simulink model "Furnace"  (R2020a)
settings: Solver=ode15s  StartTime=0  StopTime=27000  FixedStep=0.1  MaxStep=20  MinStep=1e-13  RelTol=1e-08  AbsTol=1e-09
undefined symbols (not defined in the file): agnostic_lqe_params, cont_reg, disturbance_type, F_aI_pid, F_aII_pid, input_type, k, lqe_params, LQR_params, LQRAgnostic_params, MPC_type, MPCDiscrete_function_parameters, MPCDiscreteAgnostic_function_parameters, MPCDiscreteDiffIntegralAgnostic_function_parameters, original_LQR_params, output_type, reg, single_butter_ss
libraries: simulink x35, cstblocks x10, mpclib x3
(part 7 of 8)

== matlab function Furnace/Controller/Input  selector1 ==
  data: constant input; signal output; experimental input; controlled input; input_type input
function signal = ChooseSignal(constant, experimental, controlled, input_type)
    switch(input_type)
        case InputType.Experimental
            signal = experimental;
        case InputType.Controlled
            signal = controlled;
        otherwise
            signal = constant;
    end
end

== matlab function Furnace/Controller/Input  selector2 ==
  data: constant input; signal output; experimental input; controlled input; input_type input
function signal = ChooseSignal(constant, experimental, controlled, input_type)
    switch(input_type)
        case InputType.Experimental
            signal = experimental;
        case InputType.Controlled
            signal = controlled;
        otherwise
            signal = constant;
    end
end

== matlab function Furnace/Controller/Input  selector5 ==
  data: constant input; signal output; experimental input; controlled input; input_type input
function signal = ChooseSignal(constant, experimental, controlled, input_type)
    switch(input_type)
        case InputType.Experimental
            signal = experimental;
        case InputType.Controlled
            signal = controlled;
        otherwise
            signal = constant;
    end
end

== matlab function Furnace/Actuator dynamics/Secondary air/Input  selector ==
  data: constant input; signal output; experimental input; step input; controlled input; input_type input
function signal = ChooseSignal(constant, experimental, step, controlled, input_type)
    switch(input_type)
        case InputType.Experimental
            signal = experimental;
        case InputType.Controlled
            signal = controlled;
        case InputType.Step
            signal = step; 
        otherwise
            signal = constant;
    end
end

== matlab function Furnace/Actuator dynamics/Secondary air/Input  selector1 ==
  data: constant input; signal output; experimental input; step input; controlled input; input_type input
function signal = ChooseSignal(constant, experimental, step, controlled, input_type)
    switch(input_type)
        case InputType.Experimental
            signal = experimental;
        case InputType.Controlled
            signal = controlled;
        case InputType.Step
            signal = step; 
        otherwise
            signal = constant;
    end
end

== matlab function Furnace/Actuator dynamics/Waste and Primary air/Input selector ==
  data: constant input; signal output; experimental input; controlled input; input_type input
function signal = ChooseSignal(constant, experimental, controlled, input_type)
    switch(input_type)
        case InputType.Experimental
            signal = experimental;
        case InputType.Controlled
            signal = controlled;
        otherwise
            signal = constant;
    end
end

== matlab function Furnace/Deprecated, slow loop/Furnace/Boiler/Economizer/Economizer ==
  data: Fi_fg input; F_w input; Q_ECO output; T_ECO input; T_fg2 input; cp_fg input; epsilon_ECO input; T_fg3 output; eff_HE input; cp_w input; T_ECO2 output
function [Q_ECO,T_fg3,T_ECO2] = CALC_Q_ECO(Fi_fg,F_w,T_ECO,T_fg2,cp_fg,epsilon_ECO,eff_HE, cp_w)

% This function calculates the heat exchanged in the economizer

F_fg    = sum(Fi_fg);
C_min   = cp_fg.*F_fg;
if F_w == 0 
    Q_ECO   = 0;
    T_fg3   = T_fg2;
    T_ECO2  = T_ECO;
else
    Q_ECO   = epsilon_ECO.*C_min.*(T_fg2-T_ECO);
    T_fg3   = T_fg2 - Q_ECO./(cp_fg.*F_fg);
    T_ECO2  = T_ECO + Q_ECO.*eff_HE./(cp_w.*F_w);
end
Q_ECO       = Q_ECO.*eff_HE;

== matlab function Furnace/Actuator dynamics/Waste and Primary air/Input  selector ==
  data: constant input; signal output; experimental input; step input; controlled input; input_type input
function signal = ChooseSignal(constant, experimental, step, controlled, input_type)
    switch(input_type)
        case InputType.Experimental
            signal = experimental;
        case InputType.Controlled
            signal = controlled;
        case InputType.Step
            signal = step; 
        otherwise
            signal = constant;
    end
end

== matlab function Furnace/Actuator dynamics/Waste and Primary air/Input  selector1 ==
  data: constant input; signal output; experimental input; step input; controlled input; input_type input
function signal = ChooseSignal(constant, experimental, step, controlled, input_type)
    switch(input_type)
        case InputType.Experimental
            signal = experimental;
        case InputType.Controlled
            signal = controlled;
        case InputType.Step
            signal = step; 
        otherwise
            signal = constant;
    end
end

== matlab function Furnace/Actuator dynamics/Grate speed/Input  selector ==
  data: constant input; signal output; experimental input; step input; controlled input; input_type input
function signal = ChooseSignal(constant, experimental, step, controlled, input_type)
    switch(input_type)
        case InputType.Experimental
            signal = experimental;
        case InputType.Controlled
            signal = controlled;
        case InputType.Step
            signal = step; 
        otherwise
            signal = constant;
    end
end

== matlab function Furnace/Actuator dynamics/Grate speed/Input  selector1 ==
  data: constant input; signal output; experimental input; step input; controlled input; input_type input
function signal = ChooseSignal(constant, experimental, step, controlled, input_type)
    switch(input_type)
        case InputType.Experimental
            signal = experimental;
        case InputType.Controlled
            signal = controlled;
        case InputType.Step
            signal = step; 
        otherwise
            signal = constant;
    end
end

== matlab function Furnace/Deprecated, slow loop/Furnace/Condenser/District heating heat exchanger ==
  data: F_DH input; Q_HE output; p_HP input; F_turb input; T_return input; cp_water input; epsilon_HE input; Tw_ECO output; T_district output; eff_HE input
function [Q_HE,Tw_ECO,T_district] = CALC_Q_HE(F_DH,p_HP,F_turb,T_return,cp_water,epsilon_HE,eff_HE)

% This function calculates the heat exchanged between the steam from the
% drum and the water from the district heating net
C_min   = cp_water.*F_DH;
[p_sat,T_sat,~,~,~,~] = SatWater;
T_HP    = interp1(p_sat,T_sat,p_HP,'linear','extrap');
if F_turb == 0
    Q_HE    = 0;
else 
    
    Q_HE    = epsilon_HE.*C_min.*(T_HP-T_return);
end
Tw_ECO      = T_HP;
T_district  = T_return + Q_HE./C_min;
Q_HE        = Q_HE./eff_HE;

== matlab function Furnace/Deprecated, slow loop/Furnace/Boiler/Drum/DIFF_Boiler  ==
  data: Q_EVA input; dA_dt output size=1; F_ECO input; F_SH input; T_ECO input; T_drum input; Q_cleaning input; cp_water input; dM_dt output
function [dA_dt,dM_dt]  = DIFF_Boiler(Q_EVA ,F_ECO, F_SH,T_ECO, T_drum, Q_cleaning,cp_water)

% Energy in the drum [J]
%% ENERGY BALANCE EQUATION
[~,T_sat,~,h_w,h_vap,~] = SatWater;
if T_drum < 373.15
    dA_dt   = Q_EVA - Q_cleaning;
    dM_dt   = 0;
else
    % Enthalpy of water vapor at T_drum [J/kg]
    h_steam = interp1(T_sat,h_vap,T_drum,'linear','extrap');
    % Enthalpy of water at T_drum [J/kg]
    h_water = interp1(T_sat,h_w,T_drum,'linear','extrap');
    h_ECO   = h_water - cp_water.*(T_drum-T_ECO);
    % Energy balance
    dA_dt   = Q_EVA - F_SH.*h_steam  + F_ECO.*h_ECO - Q_cleaning;
    dM_dt   = - F_SH + F_ECO;
end

== matlab function Furnace/Deprecated, slow loop/Furnace/Boiler/Drum/DIFF_Boiler_2 ==
  data: A input; T_drum output; p_amb input; T_amb input; Mw_water input; V_gas input; M_H2O input; cp_water input; V_EVA input; rho_water input; M_steel input; cp_steel input; cp_fg input; Mw_air input; p output
function [T_drum,p] = Boiler(A,p_amb,T_amb,Mw_water,V_gas,M_H2O,cp_water,V_EVA,rho_water,M_steel,cp_steel,cp_fg,Mw_air)

% This function calculates the pressure and temperature in the boiler drum
% from the total energy in the drum. The start up description should be
% changed when we know how boiler start up actually works.

%%%%%%%%%%%%%%%%%%%%%%%%%%%%%%%%%%%%%%%%%%%%%%%%%%%%%%%%%%%%%%%%%%%%%%%%%%%
% Symbol        Units       Explanation
% INPUTS:
% A             [J]         Energy stored in the boiler drum
% p_amb         [Pa]        Ambient pressure
% T_amb         [K]         Ambient temperature
% Mw_water      [kg/kmol]   Molar weight of water
% V_gas         [m3]        Volume of drum boiler initilly occupied by air
% M_H2O         [kg]        Mass of water in the boiler
% cp_water      [J/kg K]    Specific heat capacity of water
% V_EVA         [m3]        Total volume of boiler
% rho_water     [kg/m3]     Density of water
% M_steel       [kg]        Total mass of steel in the boiler
% cp_steel      [J/kg K]    Specific heat capacity of steel
% cp_fg         [J/kg K]    Specific heat capicity of fuel gasses
% Mw_air        [kg/kmol]   Molar weight of air/fuel gasses
%%%%%%%%%%%%%%%%%%%%%%%%%%%%%%%%%%%%%%%%%%%%%%%%%%%%%%%%%%%%%%%%%%%%%%%%%%%

% Energy in the drum [J]
A_en        = A;
R           = 8.314462175*1E3;
%% ENERGY BALANCE EQUATION
[p_sat,T_sat,rho_vap,h_w,h_vap,~] = SatWater;
T_drum      = fzero(@find_T,273);
if T_drum < 373.15
    p  	= p_amb;
else
    p   = interp1(T_sat,p_sat,T_drum,'linear','extrap');
end

%%%%%%%%%%%%%%%%%%%%%%%%%%%%%%%%%%%%%%%%%%%%%%%%%%%%%%%%%%%%%%%%%%%%%%%%%%%
% This subfunction finds the temperature of the drum that satisfies the
% energy balance. We assume that the cold boiler is initially filled with
% water (M_H2O) and air (which occupies the volume V_gas). The boiler has a
% valve, which is open as long as T_drum<373.15K, so that the air can be
% discharged in the atmosphere as the boiler warms up and the water
% eveporates. In this way, the pressure is mantained at p=p_amb. When
% T_drum reaches 373.15K, the valve closes and pressure builds up as the
% water starts evaporating, so that saturated water and steam are always
% present in the vessel, at the relative saturated temperature and pressure

    function Res    = find_T(X)
        T_drum      = X;
        if T_drum < 373.15
            % When T_drum<375.15K, the valve is open and p=p_amb [Pa]
            p       = p_amb;
            % The air is assumed to be saturated with water [kmol_vap/kmol]
            y_sat   = CALC_xsat(T_drum);
            % Partial pressure of water vapor [Pa]
            p_vap   = y_sat*p;
            % Specific entalphy of water at 373.15K [J/kg]
            h_w_sat = interp1(T_sat,h_w,373.15,'linear','extrap');
            % Enthalpy of water at T_drum [J/kg]
            h_water = h_w_sat - cp_water.*(373.15-T_drum);
            % Enthalpy of water vapor at T_drum [J/kg]
            h_steam = interp1(T_sat,h_vap,T_drum,'linear','extrap');
            % Vapor fraction
            x_vap   = fzero(@find_x_vap,0);
            % Moles of air in the drum [kmol]
            N_air   = (p-p_vap).*V_gas./(R.*T_drum);
            % Mass of air in the drum [kg]
            M_air   = N_air.*Mw_air;
        else
            % Enthalpy of water vapor at T_drum [J/kg]
            h_steam = interp1(T_sat,h_vap,T_drum,'linear','extrap');
            % Enthalpy of water at T_drum [J/kg]
            h_water = interp1(T_sat,h_w,T_drum,'linear','extrap');
            % Pressure of boiling water at T_drum [Pa]
            p       = interp1(T_sat,p_sat,T_drum,'linear','extrap');
            % Find the vapor fraction
            x_vap   = fzero(@find_x_vap,0);
            % No air is left in the boiler after start up
            M_air   = 0;
        end

        Res         = A_en- (M_H2O.*x_vap.*h_steam + M_H2O.*(1-x_vap).*h_water -p.*V_EVA + M_steel.*cp_steel.*(T_drum-T_amb) + M_air.*cp_fg.*(T_drum-T_amb));
    end
%%%%%%%%%%%%%%%%%%%%%%%%%%%%%%%%%%%%%%%%%%%%%%%%%%%%%%%%%%%%%%%%%%%%%%%%%%%
    function Res = find_x_vap(Y)
        x_vap   = Y;
        M_vap   = x_vap.*M_H2O;
        if T_drum < 373.15
            y_sat   = CALC_xsat(T_drum);
            p_vap   = y_sat*p_amb;
            V_vap   = V_EVA - (M_H2O-M_vap)./rho_water;
            Res     = (M_vap-p_vap.*V_vap./(R.*T_drum).*Mw_water);
        else
            % Density of saturated vapor at T_drum [kg/m3]
            rho_steam   = interp1(T_sat,rho_vap,T_drum,'linear','extrap');
            % Compressibility factor of vapor [-]
            Z_steam     = p.*Mw_water./(rho_steam.*R.*T_drum);
            % Moles of water vapor [kmol]
            N_steam     = M_H2O.*x_vap./Mw_water;
            % Pressure calculated from the vapor fraction [Pa]
            V_steam     = V_EVA-(1-x_vap).*M_H2O./rho_water;
            p2          = Z_steam.*N_steam.*R.*T_drum./V_steam;
            % p2 should be the same as p
            Res     = (p-p2);
        end
    end
end

== matlab function Furnace/Deprecated, slow loop/Furnace/Boiler/Drum/DIFF_Boiler_vap ==
  data: T_drum input; x_vap output; p input; Mw_water input; M_H2O input; V_EVA input; rho_water input
function x_vap  = Boiler_vap(T_drum,p,Mw_water,M_H2O,V_EVA,rho_water)

R           = 8.314462175*1E3;
%% ENERGY BALANCE EQUATION
x_vap = fzero(@find_x_vap,0);

%%%%%%%%%%%%%%%%%%%%%%%%%%%%%%%%%%%%%%%%%%%%%%%%%%%%%%%%%%%%%%%%%%%%%%%%%%%
    function Res    = find_x_vap(Y)
        x_vap       = Y;
        M_vap       = x_vap.*M_H2O;
        if T_drum < 373.15
            y_sat   = CALC_xsat(T_drum);
            p_vap   = y_sat*p;
            V_vap   = V_EVA - (M_H2O-M_vap)./rho_water;
            Res    = (M_vap-p_vap.*V_vap./(R.*T_drum).*Mw_water);
        else
            [~,T_sat,rho_vap,~,~,~] = SatWater;
            % Density of saturated vapor at T_drum [kg/m3]
            rho_steam   = interp1(T_sat,rho_vap,T_drum,'linear','extrap');
            % Compressibility factor of vapor [-]
            Z_steam     = p.*Mw_water./(rho_steam.*R.*T_drum);
            % Moles of water vapor [kmol]
            N_steam     = M_H2O.*x_vap./Mw_water;
            % Pressure calculated from the vapor fraction [Pa]
            V_steam     = V_EVA-(1-x_vap).*M_H2O./rho_water;
            p2          = Z_steam.*N_steam.*R.*T_drum./V_steam;
            % p2 should be the same as p
            Res         = (p-p2);
        end
    end
end
% function x  = Boiler_vap(T_drum,p,p_amb,Mw_water,V_gas,M_H2O,V_EVA,rho_water)
% 
% R           = 8.314462175*1E3;
% %% ENERGY BALANCE EQUATION
% [p_sat,T_sat,rho_vap,~,~,~] = SatWater;
% x   = fzero(@find_x_vap,0);
% 
% 
% function Res = find_x_vap(Y)
% x_vap   = Y;
% if T_drum < 373.15
%     y_sat   = CALC_xsat(T_drum);
%     p_vap   = y_sat*p_amb;
%     rho_steam = interp1(T_sat,rho_vap,T_drum,'linear','extrap');
%     p_steam = interp1(T_sat,p_sat,T_drum,'linear','extrap');
%     Z_steam = p_steam.*Mw_water./(rho_steam.*R.*T_drum);
%     M_H2O_v = p_vap.*V_gas./(Z_steam.*R.*T_drum).*Mw_water;
%     x_vap2  = M_H2O_v/M_H2O;
%     a       = (x_vap-x_vap2).*1000;
% else
%     rho_steam = interp1(T_sat,rho_vap,T_drum,'linear','extrap');
%     Z_steam = p.*Mw_water./(rho_steam.*R.*T_drum);
%     N_steam = M_H2O.*x_vap./Mw_water;
%     p_vap   = Z_steam.*N_steam.*R.*T_drum./(V_EVA-(1-x_vap).*M_H2O./rho_water);
%     a       = (p-p_vap);
% end
% Res     = a;
% end
% end

== matlab function Furnace/Deprecated, slow loop/Furnace/Free board/DIFF_Free Board ==
  data: M_fg_int input; dMfg_dt_int output; T_fg input; Fi_in input; T_in input; F_aII input; T_aII input; Q_rad input; p_amb input; dTfg_dt output; Fi_fg_out output; M_fg output; Y_H2O output; V_FreeBoard input; Mw_gas input; T_amb input; cp_fg input; cp_steel input; M_steel_FB input
function [dMfg_dt_int, dTfg_dt,Fi_fg_out,M_fg,Y_H2O] = DIFF_FreeBoard(M_fg_int,T_fg,Fi_in,T_in,F_aII,T_aII,Q_rad,p_amb,V_FreeBoard,Mw_gas,T_amb,cp_fg,cp_steel,M_steel_FB)

% This function calculates the mass and energy balance of the freeboard. The
% furnacefreaboard is treated as one control volume, where the pressure is
% assumed constant in time. 

%%%%%%%%%%%%%%%%%%%%%%%%%%%%%%%%%%%%%%%%%%%%%%%%%%%%%%%%%%%%%%%%%%%%%%%%%%
% Symbol        Units       Explanation
% INPUTS:
% M_fg_int      [kg]        Mass of gas components in the free-board (last
%                           component is missing)
% T_fg          [K]         Temperature flue gas in the free-board
% Fi_in         [kg/s]      Flue gas component mass flows from the grate
% T_in          [K]         Temperature of the flue gas from the grate
% F_aII         [kg/s]      Secondary air mass flow
% T_aII         [K]         Temperature of secondary air 
% Q_rad         [W]         Radiation heat exchanged with the grate
% k              -          Vector of constant parameters
%%%%%%%%%%%%%%%%%%%%%%%%%%%%%%%%%%%%%%%%%%%%%%%%%%%%%%%%%%%%%%%%%%%%%%%%%%

%% Parameters
R           = 8.314462175*1E3;
nc_gas      = size(Fi_in,1);

%%  FLUE GAS  
% Total amount of flue gas in the freeboard is such to have constant p (p=amb)
N_tot       = p_amb.*V_FreeBoard./(R.*T_fg);        % N_tot is used to calculate the amount of the last gas component
N_i         = [M_fg_int./Mw_gas(1:end-1);(N_tot-sum(M_fg_int./Mw_gas(1:end-1)))];  
y_fg        = N_i./N_tot;
Mw_fg       = sum(Mw_gas.*y_fg);
M_fg_tot    = Mw_fg.*N_tot;
M_fg        = N_i.*Mw_gas;
w_fg        = M_fg./M_fg_tot;
Y_H2O       = y_fg(1);

%% INPUTS (functions of time) 
% Gas from grate 
F_in        = sum(Fi_in,1);                         % [kg/s]
w_in        = zeros(size(Fi_in));                   % [kg/kg]
y_in        = zeros(size(Fi_in));
Mw_in       = zeros(size(F_in));
for i = 1:length(F_in)
    w_in(:,i)  = Fi_in(:,i)./F_in(i); 
    y_in(:,i)  = CALC_y_a(w_in(:,i),Mw_gas);        % [kmol/kmol]
    Mw_in(1,i) = sum(Mw_gas.*y_in(:,i));            % [kg/kmol]
end
Q_conv      = sum(F_in.*cp_fg.*(T_in'-T_fg));       % [W]
% Secondary air
w_aII       = CALC_w_ha(T_amb,90,Mw_gas);           % [kg/kg]
Fi_aII      = w_aII.*F_aII;                         % [kg/s]
y_aII       = CALC_y_a(w_aII,Mw_gas);               % [kmol/kmol]
Mw_aII      = sum(Mw_gas.*y_aII);                   % [K]

%% Reaction rates
R_gas       = CALC_Rw_Gas(M_fg,T_fg,nc_gas,Mw_gas,V_FreeBoard);               % [kg/s]
N_gas       = R_gas.R./Mw_gas;                      % [kmol/s]

%% Differential equations
% Temperature equation
dTfg_dt     = 1./(cp_fg.*M_fg_tot+cp_steel.*M_steel_FB).*(Q_conv+F_aII.*cp_fg.*(T_aII-T_fg)+...  	
              R_gas.H+...                                                        
              Q_rad);     
% Time derivative of gas moles in freeboard
dNfg_dt_tot = -N_tot./T_fg.*dTfg_dt;
% Total mole balance
N_out       = sum(F_in./Mw_in) + F_aII./Mw_aII + sum(N_gas) - dNfg_dt_tot;
F_fg_out    = N_out.*Mw_fg;
Fi_fg_out   = F_fg_out.*w_fg;
% Flue gas composition equation
dMfg_dt     = sum(Fi_in,2) + Fi_aII + R_gas.R - Fi_fg_out ;
dMfg_dt_int = dMfg_dt(1:end-1);

== matlab function Furnace/Deprecated, slow loop/Furnace/Gas cleaning systems/SIGURD - Slangefilter ==
  data: T_in input; T_out output; Fi_in input; Fi_solid input; F_kull input; Mw_gas input; Fi_out output; F_ashes output
function [T_out, Fi_out, F_ashes] = fcn(T_in,Fi_in,Fi_solid, F_kull,Mw_gas)


T_out   = T_in;
Fi_out  = Fi_in;
F_ashes = 0;

== matlab function Furnace/Deprecated, slow loop/Furnace/Gas cleaning systems/HeatEx 1 ==
  data: T_in input; T_out output; Fi_in input; T_damp input; epsilon input; Fi_out output; cp_fg input; Q output
function [T_out, Fi_out, Q] = fcn(T_in,Fi_in,  T_damp, epsilon,cp_fg)

% This block is already ready 

F_fg    = sum(Fi_in);
C_min   = cp_fg.*F_fg;
Q       = epsilon.*C_min.*(T_damp-T_in);
T_out   = T_in + Q./(cp_fg.*F_fg);
Fi_out  = Fi_in;

== matlab function Furnace/Deprecated, slow loop/Furnace/Gas cleaning systems/HeatEx 2 ==
  data: T_in input; T_out output; Fi_fg input; Fi_fg output; T2_in input; Fi_fg2 input; epsilon input; eff input; T2_out output; Fi_fg2 output; cp_fg input; Q_loss output
function [T_out, Fi_fg,T2_out, Fi_fg2,Q_loss] = fcn(T_in,Fi_fg, T2_in,Fi_fg2, epsilon,eff,cp_fg)

% This block is already ready 

F_fg1   = sum(Fi_fg);
F_fg2   = sum(Fi_fg2);
C_min   = cp_fg.*min(F_fg1,F_fg2);
Q       = epsilon.*C_min.*(T2_in-T_in);
T_out   = T_in + Q./(cp_fg.*F_fg1);
T2_out  = T2_in- Q./eff./(cp_fg.*F_fg2);
Q_loss  = (1-eff).*Q./eff;

== matlab function Furnace/Deprecated, slow loop/Furnace/Gas cleaning systems/HeatEx 3 ==
  data: T_in input; T_out output; Fi_fg input; T_damp input; Fi_fg output; Q output; epsilon input; cp_fg input
function [T_out, Fi_fg, Q] = fcn(T_in,Fi_fg,  T_damp,epsilon,cp_fg)

% This block is already ready 

F_fg    = sum(Fi_fg);
C_min   = cp_fg.*F_fg;
Q       = epsilon.*C_min.*(T_damp-T_in);
T_out   = T_in + Q./(cp_fg.*F_fg);

== matlab function Furnace/Deprecated, slow loop/Furnace/Gas cleaning systems/SIGURD - SCR (Katalisator) ==
  data: T_in input; T_out output; Fi_fg input; Fi_fg output; F_NH3 input; Mw_gas input
function [T_out, Fi_fg] = fcn(T_in,Fi_fg, F_NH3,Mw_gas)

%%%%%%%%%%%%%%%%%%%%%%%%%%%%%%%%%%%%%%%%%%%%%%%%%%%%%%%%%%%%%%%%%%%%%%%%%%
% INPUTS:
% T_in      [K]         Temperature of the inlet flue gas
% Fi_in     [kg/s]      Vector of mass flow of the gas components
% F_kalk    [kg/s]      Mass flow of kalk
% Mw_gas    [kg/kmol]   Vector of molar masses of the gas components

T_out   = T_in;

== matlab function Furnace/Deprecated, slow loop/Furnace/Turbine/Turbine ==
  data: T_SH input; F_SH input; p_drum input; W_el output; p_HP input; p_LP input; Q_turb output; eta_TURB input
function [W_el, Q_turb ]  = CALC_Turbine(T_SH,F_SH,p_drum,p_HP,p_LP,eta_TURB)

% This function calculates the heat exchanged in the economizer
[p_sat,T_sat,~,~,h_vap,c_p] = SatWater;
cp_vap  = interp1(p_sat,c_p,p_drum,'linear','extrap');
h_sat   = interp1(p_sat,h_vap,p_drum,'linear','extrap');
T_drum  = interp1(p_sat,T_sat,p_drum,'linear','extrap');
h_in    = h_sat + cp_vap.*(T_SH - T_drum);
h_HP    = interp1(p_sat,h_vap,p_HP,'linear','extrap');
% h_LP    = interp1(p_sat,h_vap,p_LP,'linear','extrap');
Q_in    = F_SH.*(h_in - h_HP);
W_el    = eta_TURB.*Q_in;
Q_turb  = (1-eta_TURB).*Q_in;

% % This function calculates the heat exchanged in the economizer
% [p_sat,T_sat,~,~,h_vap,c_p] = SatWater;
% cp_vap  = interp1(p_sat,c_p,p_drum,'linear','extrap');
% h_sat   = interp1(p_sat,h_vap,p_drum,'linear','extrap');
% T_drum  = interp1(p_sat,T_sat,p_drum,'linear','extrap');
% h_in    = h_sat + cp_vap.*(T_SH - T_drum);
% Q_in    = F_SH.*(cp_vap.*(T_SH-T_cond) - H_eva);
% eta_TURB= 32.74 - 0.026.*(T_toDH - 273.15) - 0.089.*(T_fromDH - 273.15);
% W_el    = eta_TURB.*Q_in./100;
% T_turb  = T_cond;

== matlab function Furnace/Deprecated, slow loop/Furnace/Gas cleaning systems/HeatEx 4 ==
  data: T_in input; T_out output; Fi_fg input; Fi_fg output; T2_in input; Fi_fg2 input; epsilon input; T2_out output; Fi_fg2 output; cp_fg input
function [T_out, Fi_fg,T2_out, Fi_fg2] = fcn(T_in,Fi_fg, T2_in,Fi_fg2, epsilon,cp_fg)


F_fg1   = sum(Fi_fg);
F_fg2   = sum(Fi_fg2);
C_min   = cp_fg.*min(F_fg1,F_fg2);
Q       = epsilon.*C_min.*(T_in-T2_in);
T_out   = T_in - Q./(cp_fg.*F_fg1);
T2_out  = T2_in+ Q./(cp_fg.*F_fg2);

== matlab function Furnace/Deprecated, slow loop/Furnace/Gas cleaning systems/SIGURD - Scrubber ==
  data: T_in input; T_out output; Fi_in input; Fi_out output; F_NH3 input; Mw_gas input
function [T_out, Fi_out] = fcn(T_in,Fi_in, F_NH3,Mw_gas)

%%%%%%%%%%%%%%%%%%%%%%%%%%%%%%%%%%%%%%%%%%%%%%%%%%%%%%%%%%%%%%%%%%%%%%%%%%
% INPUTS:
% T_in      [K]         Temperature of the inlet flue gas
% Fi_in     [kg/s]      Vector of mass flow of the gas components
% F_kalk    [kg/s]      Mass flow of kalk
% Mw_gas    [kg/kmol]   Vector of molar masses of the gas components


T_out   = T_in;
Fi_out  = Fi_in;

== matlab function Furnace/Deprecated, slow loop/Furnace/Flue-gas fan/Fan ==
  data: T_fg input; T_out output; F_fg input; W_el output
function [T_out, W_el] = fcn(T_fg,F_fg)

T_out = T_fg;
W_el = 0;

== matlab function Furnace/Deprecated, slow loop/Controller/Summer Controller (Cleaned)/Controller selector  ==
  data: ab input; cascade input; signal output; mpc input; controller_type input
function signal = ChooseController(ab, cascade, mpc, controller_type)
   
switch(controller_type)
        case ControllerType.AB
            signal = ab;
        case ControllerType.Cascade
            signal = cascade;
        otherwise
            signal = mpc;
    end
end

== matlab function Furnace/Deprecated, slow loop/Controller/Summer Controller (Cleaned)/Controller selector 1 ==
  data: ab input; cascade input; signal output; mpc input; controller_type input
function signal = ChooseController(ab, cascade, mpc, controller_type)
   
switch(controller_type)
        case ControllerType.AB
            signal = ab;
        case ControllerType.Cascade
            signal = cascade;
        otherwise
            signal = mpc;
    end
end

== matlab function Furnace/Deprecated, slow loop/Furnace/Boiler/MATLAB Function ==
  data: p_drum input; k_p_drum input; switch_on output
function switch_on = calc_swch(p_drum, k_p_drum)

switch_on = 0;
if p_drum >= k_p_drum
    switch_on = 1;
end

== matlab function Furnace/Deprecated, slow loop/Controller/Summer Controller (Cleaned)/Controller selector 2 ==
  data: ab input; cascade input; signal output; mpc input; controller_type input
function signal = ChooseController(ab, cascade, mpc, controller_type)
   
switch(controller_type)
        case ControllerType.AB
            signal = ab;
        case ControllerType.Cascade
            signal = cascade;
        otherwise
            signal = mpc;
    end
end

== matlab function Furnace/Deprecated, slow loop/Controller/Summer Controller (Cleaned)/Controller selector 3 ==
  data: ab input; cascade input; signal output; mpc input; controller_type input
function signal = ChooseController(ab, cascade, mpc, controller_type)
   
switch(controller_type)
        case ControllerType.AB
            signal = ab;
        case ControllerType.Cascade
            signal = cascade;
        otherwise
            signal = mpc;
    end
end

== matlab function Furnace/Plant2/Boiler/Drum/DIFF_Boiler  ==
  data: Q_EVA input; dA_dt output size=1; F_ECO input; F_SH input; T_ECO input; T_drum input; Q_cleaning input; cp_water input; dM_dt output
function [dA_dt,dM_dt]  = DIFF_Boiler(Q_EVA ,F_ECO, F_SH,T_ECO, T_drum, Q_cleaning,cp_water)

% Energy in the drum [J]
%% ENERGY BALANCE EQUATION
[~,T_sat,~,h_w,h_vap,~] = SatWater;
if T_drum < 373.15
    dA_dt   = Q_EVA - Q_cleaning;
    dM_dt   = 0;
else
    % Enthalpy of water vapor at T_drum [J/kg]
    h_steam = interp1(T_sat,h_vap,T_drum,'linear','extrap');
    % Enthalpy of water at T_drum [J/kg]
    h_water = interp1(T_sat,h_w,T_drum,'linear','extrap');
    h_ECO   = h_water - cp_water.*(T_drum-T_ECO);
    % Energy balance
    dA_dt   = Q_EVA - F_SH.*h_steam  + F_ECO.*h_ECO - Q_cleaning;
    dM_dt   = - F_SH + F_ECO;
end

== matlab function Furnace/Plant2/Boiler/Drum/DIFF_Boiler_2 ==
  data: A input; T_drum output; p_amb input; T_amb input; Mw_water input; V_gas input; M_H2O input; cp_water input; V_EVA input; rho_water input; M_steel input; cp_steel input; cp_fg input; Mw_air input; p output
function [T_drum,p] = Boiler(A,p_amb,T_amb,Mw_water,V_gas,M_H2O,cp_water,V_EVA,rho_water,M_steel,cp_steel,cp_fg,Mw_air)

% This function calculates the pressure and temperature in the boiler drum
% from the total energy in the drum. The start up description should be
% changed when we know how boiler start up actually works.

%%%%%%%%%%%%%%%%%%%%%%%%%%%%%%%%%%%%%%%%%%%%%%%%%%%%%%%%%%%%%%%%%%%%%%%%%%%
% Symbol        Units       Explanation
% INPUTS:
% A             [J]         Energy stored in the boiler drum
% p_amb         [Pa]        Ambient pressure
% T_amb         [K]         Ambient temperature
% Mw_water      [kg/kmol]   Molar weight of water
% V_gas         [m3]        Volume of drum boiler initilly occupied by air
% M_H2O         [kg]        Mass of water in the boiler
% cp_water      [J/kg K]    Specific heat capacity of water
% V_EVA         [m3]        Total volume of boiler
% rho_water     [kg/m3]     Density of water
% M_steel       [kg]        Total mass of steel in the boiler
% cp_steel      [J/kg K]    Specific heat capacity of steel
% cp_fg         [J/kg K]    Specific heat capicity of fuel gasses
% Mw_air        [kg/kmol]   Molar weight of air/fuel gasses
%%%%%%%%%%%%%%%%%%%%%%%%%%%%%%%%%%%%%%%%%%%%%%%%%%%%%%%%%%%%%%%%%%%%%%%%%%%

% Energy in the drum [J]
A_en        = A;
R           = 8.314462175*1E3;
%% ENERGY BALANCE EQUATION
[p_sat,T_sat,rho_vap,h_w,h_vap,~] = SatWater;
T_drum      = fzero(@find_T,273);
if T_drum < 373.15
    p  	= p_amb;
else
    p   = interp1(T_sat,p_sat,T_drum,'linear','extrap');
end

%%%%%%%%%%%%%%%%%%%%%%%%%%%%%%%%%%%%%%%%%%%%%%%%%%%%%%%%%%%%%%%%%%%%%%%%%%%
% This subfunction finds the temperature of the drum that satisfies the
% energy balance. We assume that the cold boiler is initially filled with
% water (M_H2O) and air (which occupies the volume V_gas). The boiler has a
% valve, which is open as long as T_drum<373.15K, so that the air can be
% discharged in the atmosphere as the boiler warms up and the water
% eveporates. In this way, the pressure is mantained at p=p_amb. When
% T_drum reaches 373.15K, the valve closes and pressure builds up as the
% water starts evaporating, so that saturated water and steam are always
% present in the vessel, at the relative saturated temperature and pressure

    function Res    = find_T(X)
        T_drum      = X;
        if T_drum < 373.15
            % When T_drum<375.15K, the valve is open and p=p_amb [Pa]
            p       = p_amb;
            % The air is assumed to be saturated with water [kmol_vap/kmol]
            y_sat   = CALC_xsat(T_drum);
            % Partial pressure of water vapor [Pa]
            p_vap   = y_sat*p;
            % Specific entalphy of water at 373.15K [J/kg]
            h_w_sat = interp1(T_sat,h_w,373.15,'linear','extrap');
            % Enthalpy of water at T_drum [J/kg]
            h_water = h_w_sat - cp_water.*(373.15-T_drum);
            % Enthalpy of water vapor at T_drum [J/kg]
            h_steam = interp1(T_sat,h_vap,T_drum,'linear','extrap');
            % Vapor fraction
            x_vap   = fzero(@find_x_vap,0);
            % Moles of air in the drum [kmol]
            N_air   = (p-p_vap).*V_gas./(R.*T_drum);
            % Mass of air in the drum [kg]
            M_air   = N_air.*Mw_air;
        else
            % Enthalpy of water vapor at T_drum [J/kg]
            h_steam = interp1(T_sat,h_vap,T_drum,'linear','extrap');
            % Enthalpy of water at T_drum [J/kg]
            h_water = interp1(T_sat,h_w,T_drum,'linear','extrap');
            % Pressure of boiling water at T_drum [Pa]
            p       = interp1(T_sat,p_sat,T_drum,'linear','extrap');
            % Find the vapor fraction
            x_vap   = fzero(@find_x_vap,0);
            % No air is left in the boiler after start up
            M_air   = 0;
        end

        Res         = A_en- (M_H2O.*x_vap.*h_steam + M_H2O.*(1-x_vap).*h_water -p.*V_EVA + M_steel.*cp_steel.*(T_drum-T_amb) + M_air.*cp_fg.*(T_drum-T_amb));
    end
%%%%%%%%%%%%%%%%%%%%%%%%%%%%%%%%%%%%%%%%%%%%%%%%%%%%%%%%%%%%%%%%%%%%%%%%%%%
    function Res = find_x_vap(Y)
        x_vap   = Y;
        M_vap   = x_vap.*M_H2O;
        if T_drum < 373.15
            y_sat   = CALC_xsat(T_drum);
            p_vap   = y_sat*p_amb;
            V_vap   = V_EVA - (M_H2O-M_vap)./rho_water;
            Res     = (M_vap-p_vap.*V_vap./(R.*T_drum).*Mw_water);
        else
            % Density of saturated vapor at T_drum [kg/m3]
            rho_steam   = interp1(T_sat,rho_vap,T_drum,'linear','extrap');
            % Compressibility factor of vapor [-]
            Z_steam     = p.*Mw_water./(rho_steam.*R.*T_drum);
            % Moles of water vapor [kmol]
            N_steam     = M_H2O.*x_vap./Mw_water;
            % Pressure calculated from the vapor fraction [Pa]
            V_steam     = V_EVA-(1-x_vap).*M_H2O./rho_water;
            p2          = Z_steam.*N_steam.*R.*T_drum./V_steam;
            % p2 should be the same as p
            Res     = (p-p2);
        end
    end
end

== matlab function Furnace/Deprecated, slow loop/Furnace/Gas cleaning systems/SIGURD - Reaktor ==
  data: T_in input; T_out output; Fi_in input; F_flyash input; Fi_out output; F_kalk input; Mw_gas input; cp_fg input; F_solid output; F_H2O input
function [T_out, Fi_out, F_solid] = fcn(T_in,Fi_in, F_flyash,F_kalk,Mw_gas,cp_fg, F_H2O)

%%%%%%%%%%%%%%%%%%%%%%%%%%%%%%%%%%%%%%%%%%%%%%%%%%%%%%%%%%%%%%%%%%%%%%%%%%
% INPUTS:
% T_in      [K]         Temperature of the inlet flue gas
% Fi_in     [kg/s]      Vector of mass flow of the gas components
% F_kalk    [kg/s]      Mass flow of kalk
% Mw_gas    [kg/kmol]   Vector of molar masses of the gas components


T_out   = T_in;
Fi_out  = Fi_in;
% The total amount of solid particles equals the flow of flyashes that 
% follow the gas from the combustion chamber + the solid phase particles 
% that form in the reactor
F_solid = F_flyash + 0;

== matlab function Furnace/Deprecated, slow loop/Controller/Summer Controller (Cleaned)/Input  selector2 ==
  data: constant input; signal output; experimental input; controlled input; input_type input
function signal = ChooseSignal(constant, experimental, controlled, input_type)
    switch(input_type)
        case InputType.Experimental
            signal = experimental;
        case InputType.Controlled
            signal = controlled;
        otherwise
            signal = constant;
    end
end

== matlab function Furnace/Deprecated, slow loop/Controller/Summer Controller (Old) /Input  selector1 ==
  data: constant input; signal output; experimental input; controlled input; input_type input
function signal = ChooseSignal(constant, experimental, controlled, input_type)
    switch(input_type)
        case InputType.Experimental
            signal = experimental;
        case InputType.Controlled
            signal = controlled;
        otherwise
            signal = constant;
    end
end

== matlab function Furnace/Deprecated, slow loop/Controller/Summer Controller (Old) /Input  selector ==
  data: constant input; signal output; experimental input; controlled input; input_type input
function signal = ChooseSignal(constant, experimental, controlled, input_type)
    switch(input_type)
        case InputType.Experimental
            signal = experimental;
        case InputType.Controlled
            signal = controlled;
        otherwise
            signal = constant;
    end
end

== matlab function Furnace/Deprecated, slow loop/Controller/Summer Controller (Old) /Controller selector  ==
  data: ab input; cascade input; signal output; mpc input; controller_type input
function signal = ChooseController(ab, cascade, mpc, controller_type)
   
switch(controller_type)
        case ControllerType.AB
            signal = ab;
        case ControllerType.Cascade
            signal = cascade;
        otherwise
            signal = mpc;
    end
end

== matlab function Furnace/Deprecated, slow loop/Controller/Summer Controller (Old) /Controller selector 1 ==
  data: ab input; cascade input; signal output; mpc input; controller_type input
function signal = ChooseController(ab, cascade, mpc, controller_type)
   
switch(controller_type)
        case ControllerType.AB
            signal = ab;
        case ControllerType.Cascade
            signal = cascade;
        otherwise
            signal = mpc;
    end
end

== matlab function Furnace/Deprecated, slow loop/Controller/Summer Controller (Old) /Controller selector 2 ==
  data: ab input; cascade input; signal output; mpc input; controller_type input
function signal = ChooseController(ab, cascade, mpc, controller_type)
   
switch(controller_type)
        case ControllerType.AB
            signal = ab;
        case ControllerType.Cascade
            signal = cascade;
        otherwise
            signal = mpc;
    end
end

== matlab function Furnace/Deprecated, slow loop/Controller/Summer Controller (Old) /Controller selector 3 ==
  data: ab input; cascade input; signal output; mpc input; controller_type input
function signal = ChooseController(ab, cascade, mpc, controller_type)
   
switch(controller_type)
        case ControllerType.AB
            signal = ab;
        case ControllerType.Cascade
            signal = cascade;
        otherwise
            signal = mpc;
    end
end

== matlab function Furnace/Deprecated, slow loop/Furnace/Calorific Value/MATLAB Function ==
  data: Fi_fg input; HHV output; T_fg input; cp_fg input; T_amb input; F_aI input; T_aI input; F_aII input; T_aII input
function HHV = CalorificValue(Fi_fg,T_fg,cp_fg,T_amb,F_aI,T_aI,F_aII,T_aII)

HHV = sum(Fi_fg).*cp_fg.*(T_fg-T_amb);%-sum(F_aI).*cp_fg.*(T_aI-T_amb)-F_aII.*cp_fg.*(T_aII-T_amb);

== matlab function Furnace/Deprecated, slow loop/Controller/Summer Controller (Cleaned)/Input  selector3 ==
  data: constant input; signal output; experimental input; controlled input; input_type input
function signal = ChooseSignal(constant, experimental, controlled, input_type)
    switch(input_type)
        case InputType.Experimental
            signal = experimental;
        case InputType.Controlled
            signal = controlled;
        otherwise
            signal = constant;
    end
end

== matlab function Furnace/Deprecated, slow loop/Controller/Summer Controller (Old) /Input  selector3 ==
  data: constant input; signal output; experimental input; controlled input; input_type input
function signal = ChooseSignal(constant, experimental, controlled, input_type)
    switch(input_type)
        case InputType.Experimental
            signal = experimental;
        case InputType.Controlled
            signal = controlled;
        otherwise
            signal = constant;
    end
end

== matlab function Furnace/Deprecated, slow loop/Controller/Summer Controller (Old) /Input  selector4 ==
  data: constant input; signal output; experimental input; controlled input; input_type input
function signal = ChooseSignal(constant, experimental, controlled, input_type)
    switch(input_type)
        case InputType.Experimental
            signal = experimental;
        case InputType.Controlled
            signal = controlled;
        otherwise
            signal = constant;
    end
end

== matlab function Furnace/Deprecated, slow loop/Controller/Summer Controller (Old) /Input  selector5 ==
  data: constant input; signal output; experimental input; controlled input; input_type input
function signal = ChooseSignal(constant, experimental, controlled, input_type)
    switch(input_type)
        case InputType.Experimental
            signal = experimental;
        case InputType.Controlled
            signal = controlled;
        otherwise
            signal = constant;
    end
end

== matlab function Furnace/Deprecated, slow loop/Controller/Summer Controller (Old) /Input  selector2 ==
  data: constant input; signal output; experimental input; controlled input; input_type input
function signal = ChooseSignal(constant, experimental, controlled, input_type)
    switch(input_type)
        case InputType.Experimental
            signal = experimental;
        case InputType.Controlled
            signal = controlled;
        otherwise
            signal = constant;
    end
end

== matlab function Furnace/Deprecated, slow loop/Contineous Summer student feedback (Not finished)/Controller/Controller selector  ==
  data: ab input; cascade input; signal output; mpc input; controller_type input
function signal = ChooseController(ab, cascade, mpc, controller_type)
   
switch(controller_type)
        case ControllerType.AB
            signal = ab;
        case ControllerType.Cascade
            signal = cascade;
        otherwise
            signal = mpc;
    end
end

== matlab function Furnace/Deprecated, slow loop/Contineous Summer student feedback (Not finished)/Controller/Controller selector 1 ==
  data: ab input; cascade input; signal output; mpc input; controller_type input
function signal = ChooseController(ab, cascade, mpc, controller_type)
   
switch(controller_type)
        case ControllerType.AB
            signal = ab;
        case ControllerType.Cascade
            signal = cascade;
        otherwise
            signal = mpc;
    end
end

== matlab function Furnace/Deprecated, slow loop/Furnace/Grate/Diff_Grate ==
  data: M_w input; dMw_dt_col output; T_w input; M_char input; Fi_w_in input; T_w_in input; F_aI input; T_aI input; Q_rad input; Q_burners input; Q_grate input; v_grate input; L input; Delta_H input; cp_w input; cp_steel input; M_steel_grate input; cp_fg input; Mw_w input; Mw_gas input; p_amb input; T_amb input; k_w input; k_grate input; W input; rho_w input; A_grate input; dTw_dt_col output; dMchar_dt_col output; F_fg_out output; F_flyash output; F_w_ash output; F_char_ash output; t input
function [dMw_dt_col,dTw_dt_col,dMchar_dt_col,F_fg_out,F_flyash,F_w_ash,F_char_ash]= DIFF_Grate(M_w,T_w,M_char,Fi_w_in,T_w_in,F_aI,T_aI,Q_rad,Q_burners,Q_grate,v_grate,L,Delta_H,cp_w,cp_steel,M_steel_grate,cp_fg,Mw_w,Mw_gas,p_amb,T_amb,k_w,k_grate,W,rho_w,A_grate,t)

% This function calculates the mass and energy balance of the furnace. The
% furnace is treated as a one dimensional system, which is discretized in
% 'n_cell'-control volumes, in the direction of movement of the waste on 
% the grate.

%%%%%%%%%%%%%%%%%%%%%%%%%%%%%%%%%%%%%%%%%%%%%%%%%%%%%%%%%%%%%%%%%%%%%%%%%%
% Symbol        Units       Explanation
% INPUTS:
% M_w           [kg]        Mass of waste components in each cell of the furnace
% T_w           [K]         Temperature of waste in each cell ot the furnace
% M_char        [kg]        Mass char in each cell of the furnace
% Fi_w_in       [kg/s]      Waste component mass flows into the furnace (it
%                           enters the first cell of the furnace.
% T_w_in        [K]         Temperature of the waste entering the furnace
% F_aI          [kg/s]      Primary air component mass flows in each zone
%                           (there are 'n_zone'-zones)
% T_aI          [K]         Temperature of primary air (same in every zone)
% Q_rad         [W]         Radiative heat to each cell
% Q_burners     [W]         Toatal heat delivered by auxiliary burners
% Q_grate       [W]         Heat removed by grate cooling (only zones 1-3)
% k              -          Vector of constant parameters
% t             [s]         Time 
%%%%%%%%%%%%%%%%%%%%%%%%%%%%%%%%%%%%%%%%%%%%%%%%%%%%%%%%%%%%%%%%%%%%%%%%%%

%% SOLID WASTE 
T_w         = T_w';
M_char      = M_char';
n_cell      = length(T_w);
nc_w        = length(M_w)./n_cell;
M_w         = reshape(M_w,[nc_w,n_cell]);   % Transform vector M_w into a matrix
Mw_tot      = sum(M_w,1) + M_char;          % Total mass in each zone [kg]

%% GEOMETRTICAL GRID
n_zone      = length(F_aI);
L_zone      = L./n_zone;                    % [m]
L_cell      = L./n_cell;                    % [m]
n           = 50;
x_zone      = linspace(0,L,n*n_zone);
x_cell      = linspace(0,L,n*n_cell);
F_aI_x      = zeros(size(x_zone));
T_aI_x      = zeros(size(x_zone));
Q_grate_x   = zeros(size(x_zone));
if Q_burners > 0
    Q_grate = zeros(5,1);                   % No grate cooling when the burners are on
else 
    Q_grate = [Q_grate; 0; 0];              % There is no grate cooling in zone 4 and 5
end
for i=1:n_zone
    F_aI_x((i-1)*n+1:i*n)   = F_aI(i).*ones(1,n)./L_zone;
    T_aI_x((i-1)*n+1:i*n)   = T_aI.*ones(1,n);
    Q_grate_x((i-1)*n+1:i*n)= Q_grate(i).*ones(1,n)./L_zone;
end
F_aI_dx     = interp1(x_zone,F_aI_x,x_cell);
T_aI_dx     = interp1(x_zone,T_aI_x,x_cell);
Q_grate_dx  = interp1(x_zone,Q_grate_x,x_cell);
F_aI        = zeros(size(T_w));
T_aI        = zeros(size(T_w));
Q_grate     = zeros(size(T_w));

for i = 1:n_cell
    F_aI(1,i)   = trapz(x_cell((i-1)*n+1:i*n),F_aI_dx((i-1)*n+1:i*n));
    T_aI(1,i)   = trapz(x_cell((i-1)*n+1:i*n),F_aI_dx((i-1)*n+1:i*n).*T_aI_dx((i-1)*n+1:i*n))./F_aI(1,i);
    Q_grate(1,i)= trapz(x_cell((i-1)*n+1:i*n),Q_grate_dx((i-1)*n+1:i*n));
end
%% INPUTS 
% Flows and temperature of the waste leaving each cell
Fi_w_out    = zeros(size(M_w));
for i = 1:n_cell
    if t>=(i*L_cell/v_grate)
        Fi_w_out(:,i) = v_grate.*M_w(:,i)./L_cell;
    end
end
T_w_out     = [T_w(:,2:end) T_w(end)];
% Flows and temperature of the waste entering each cell
Fi_w_in     = [Fi_w_in, Fi_w_out(:,1:end-1)];
F_w_in      = sum(Fi_w_in,1);
T_w_in      = [T_w_in, T_w(:,1:end-1)];
% Primary air  
w_aI        = CALC_w_ha(T_amb,90,Mw_gas);
Fi_aI       = zeros(length(w_aI),length(T_w));
for i = 1:n_cell
    Fi_aI(:,i)  = w_aI(:,1).*F_aI(i);
end

%% CONDUCTION TERMS
h_w         = sum(M_w,1)./(rho_w.*W);  % the height of the waste is a function of the mass on the grate
A_w         = W.*h_w;
% Conduction heat through the waste layer
Q_cond_w_in = -k_w.*A_w.*(T_w-T_w_in)./L_cell;
Q_cond_w_out= [Q_cond_w_in(2:end), 0];
Q_cond_w_l = [0 -k_w.*A_w(2:end).*(T_w(2:end)-T_w_in(2:end))./L_cell];
Q_cond_w_r= [Q_cond_w_l(2:end), 0];
% Conduction heat through the metal grate
Q_cond_g_in = -k_grate.*A_grate.*(T_w-T_w_in)./L_cell;
Q_cond_g_out= -k_grate.*A_grate.*(T_w_out-T_w)./L_cell;
Q_cond_g_l = [0 -k_grate.*A_grate.*(T_w(2:end)-T_w_in(2:end))./L_cell];
Q_cond_g_r= [Q_cond_g_l(2:end), 0];
% Total conduction term for each cell 
Q_cond      = Q_cond_w_l - Q_cond_w_r + Q_cond_g_l - Q_cond_g_r;

%% BURNERS
Q_burn      = Q_burners./n_cell.*ones(1,n_cell);

%% REACTION RATES
R_w         = CALC_Rw_Char(M_w,T_w,M_char,Fi_aI,Mw_w,Mw_gas,p_amb);  

%% STATIONARY TOTAL GAS BALANCE
F_fg_out    = Fi_aI + R_w.gas;
F_flyash    = -R_w.waste_cons(end,:);

%% DIFFERENTIAL EQUATIONS
% Solid waste mass balance
F_reac      = R_w.waste_cons;
dMw_dt      = Fi_w_in - Fi_w_out + F_reac;
         
% Char mass balance
F_char_out  = v_grate.*M_char./L_cell;          % [kg/s]
F_char_in   = [0, F_char_out(:,1:end-1)];
F_char_reac = R_w.char + R_w.char_cons;
dMchar_dt   = F_char_in - F_char_out + F_char_reac;       

% Enargy balance
Delta_H_tot = -(R_w.waste_cons(1,:).*Delta_H(1) + ...
                sum(R_w.waste_cons(2:end-1,:)).*Delta_H(2) + ...
                R_w.char_cons.*Delta_H(3) );
dTw_dt      = 1./(cp_w.*Mw_tot +cp_steel.*M_steel_grate./n_cell).*((F_w_in+F_char_in).*cp_w.*(T_w_in-T_w)+F_aI.*cp_fg.*(T_aI-T_w)+...  	% Convective terms
              Delta_H_tot+...                                                                                   % Reaction term
              Q_rad' +...                                                                                       % Radiation term
              Q_cond +...                                                                                       % Conduction term
              Q_burn -...                                                                                       % Burners
              Q_grate);                                                                                         % Grate cooling
% Make outputs into colums
dMw_dt_col   = reshape(dMw_dt,[n_cell*nc_w,1]);
dMchar_dt_col= dMchar_dt';
dTw_dt_col   = dTw_dt';
F_w_ash      = Fi_w_out(end+1-nc_w:end);
F_char_ash   = F_char_out(end);

== matlab function Furnace/Deprecated, slow loop/Contineous Summer student feedback (Not finished)/Controller/Controller selector 2 ==
  data: ab input; cascade input; signal output; mpc input; controller_type input
function signal = ChooseController(ab, cascade, mpc, controller_type)
   
switch(controller_type)
        case ControllerType.AB
            signal = ab;
        case ControllerType.Cascade
            signal = cascade;
        otherwise
            signal = mpc;
    end
end

== matlab function Furnace/Deprecated, slow loop/Contineous Summer student feedback (Not finished)/Controller/Controller selector 3 ==
  data: ab input; cascade input; signal output; mpc input; controller_type input
function signal = ChooseController(ab, cascade, mpc, controller_type)
   
switch(controller_type)
        case ControllerType.AB
            signal = ab;
        case ControllerType.Cascade
            signal = cascade;
        otherwise
            signal = mpc;
    end
end

== matlab function Furnace/Deprecated, slow loop/Contineous Summer student feedback (Not finished)/Controller/Input  selector ==
  data: constant input; signal output; experimental input; controlled input; input_type input
function signal = ChooseSignal(constant, experimental, controlled, input_type)
    switch(input_type)
        case InputType.Experimental
            signal = experimental;
        case InputType.Controlled
            signal = controlled;
        otherwise
            signal = constant;
    end
end

== matlab function Furnace/Deprecated, slow loop/Contineous Summer student feedback (Not finished)/Controller/Input  selector1 ==
  data: constant input; signal output; experimental input; controlled input; input_type input
function signal = ChooseSignal(constant, experimental, controlled, input_type)
    switch(input_type)
        case InputType.Experimental
            signal = experimental;
        case InputType.Controlled
            signal = controlled;
        otherwise
            signal = constant;
    end
end
